simulink model "RST_model"  (R2025a)
settings: Solver=VariableStepAuto  StartTime=0.0  StopTime=10.0  RelTol=1e-3
values from neighbouring files (symbols this model uses):
  A = Gp.Denominator{1,1}    [d5_RST.m]    (also in d5_a_1.m = Gpk.Denominator{1,1}; d5_a_2.m = Gpk.Denominator{1,1}; d5_b_1.m = Gpd.Denominator{1,1})
  B = Gp.Numerator{1,1}    [d5_RST.m]    (also in d5_a_1.m = Gpk.Numerator{1,1}; d5_a_2.m = Gpk.Numerator{1,1}; d5_b_1.m = Gpd.Numerator{1,1})
  R = double(RS(1:n))    [calculateRS.m]    (also in d5_b_2.m = (1 - 2 * c * z^(-1) + z^(-2)) / (s * z^(-1)) * R0)
  S = double(RS(n+1:end))    [calculateRS.m]    (also in d5_b_2.m = tf(double([sol.s3, sol.s2, sol.s1, sol.s0]), 1, Ts))
  T = 1 / dcgain(1 / Rs * feedback(Gp, Ss / Rs))    [d5_RST.m]    (also in d5_b_2.m = 1 / dcgain(minreal(1 / R * feedback(Gpd, S / R), 1e-2)))
settings Model: Creator=Korisnik  LastModifiedBy=Korisnik

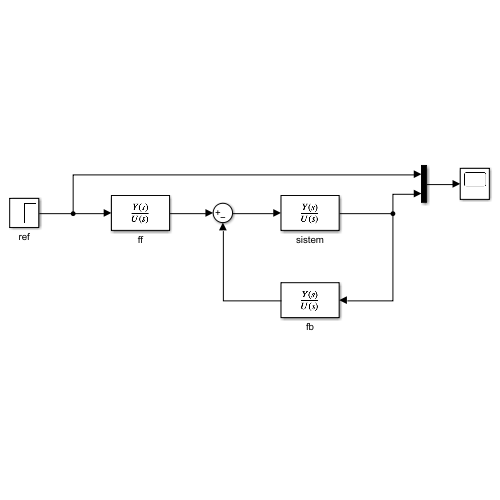
[thumbnail: Simulink's stored preview of the top-level diagram]
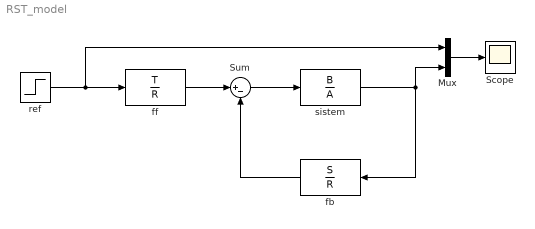
== system RST_model ==
  Mux : Mux  Inputs=2
  Scope : Scope
      settings: ActiveDisplayYMinimum=-0.37683323741197089  ActiveDisplayYMaximum=3.3914991367077389
  Sum : Sum  Inputs=|+-
  fb : TransferFcn  Numerator=S  Denominator=R
  ff : TransferFcn  Numerator=T  Denominator=R
  ref : Step  Time=0  After=3  SampleTime=0
  sistem : TransferFcn  Numerator=B  Denominator=A
  wires:
  ref/1 -> Mux/1, ff/1
  ff/1 -> Sum/1
  Sum/1 -> sistem/1
  fb/1 -> Sum/2
  sistem/1 -> Mux/2, fb/1
  Mux/1 -> Scope/1
